simulink model "Fixed_Wing_Aircraft_Sim_closed_loop"  (R2023b)
settings: Solver=ode15s  StartTime=0.0  StopTime=10000  MinStep=1e-200  RelTol=1e-3
InitFcn:
  | parameters
undefined symbols (not defined in the file or in its folder): drawAircraft, plotmavstatevariables
settings Model: Creator=Pravin  LastModifiedBy=yizho
settings SolverCC: AlgebraicLoopSolver=TrustRegion
settings DataIOCC: ReturnWorkspaceOutputs=off
settings DebuggingCC: UnconnectedInputMsg=warning  UnconnectedOutputMsg=warning  UnconnectedLineMsg=warning  ArithmeticOperatorsInVariantConditions=warning
settings ModelReferenceCC: EnableRefExpFcnMdlSchedulingChecks=on
settings SFSimCC: SimUseLocalCustomCode=off  CustomCodeUndefinedFunction=UseInterfaceOnly
settings RTWCC: RTWUseLocalCustomCode=off  DLArmComputeVersion=19.05
settings CodeAppCC: StateflowObjectComments=on

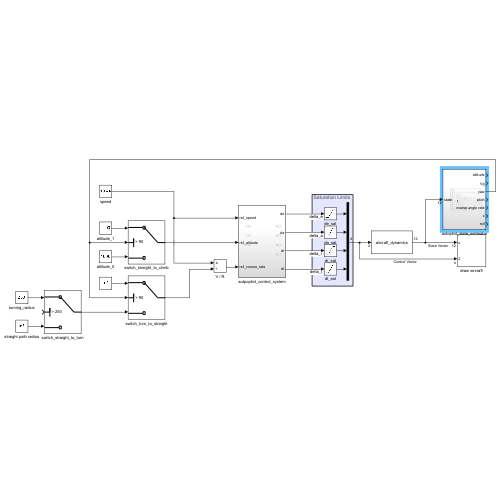
[thumbnail: Simulink's stored preview of the top-level diagram]
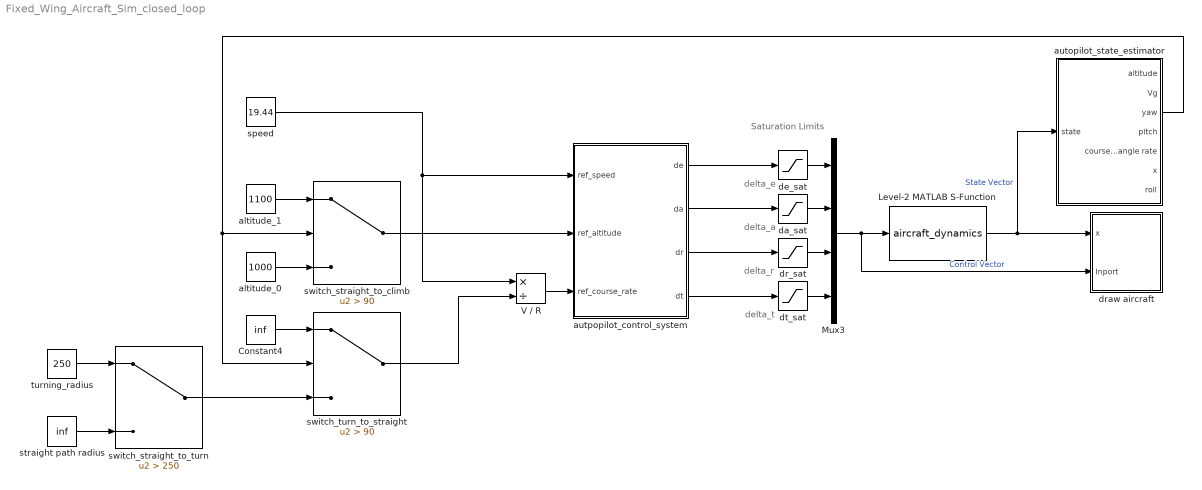
== system Fixed_Wing_Aircraft_Sim_closed_loop ==
  note: Saturation Limits
  note: delta_t
  note: delta_a
  note: delta_r
  note: delta_e
  Constant4 : Constant  Value=inf
  Level-2 MATLAB S-Function : M-S-Function  FunctionName=aircraft_dynamics  Parameters=P
  Mux3 : Mux
  V / R : Product  Inputs=*/
  altitude_0 : Constant  Value=1000
  altitude_1 : Constant  Value=1100
  autopilot_state_estimator : Subsystem
  autpopilot_control_system : Subsystem
  da_sat : Saturate  UpperLimit=50  LowerLimit=-50
  de_sat : Saturate  UpperLimit=50  LowerLimit=-50
  dr_sat : Saturate  UpperLimit=50  LowerLimit=-50
  draw aircraft : Subsystem
  dt_sat : Saturate  UpperLimit=1  LowerLimit=0
  speed : Constant  Value=19.44
  straight path radius : Constant  Value=inf
  switch_straight_to_climb : Switch  Criteria=u2 > Threshold  Threshold=90  SaturateOnIntegerOverflow=off  InputSameDT=off
  switch_straight_to_turn : Switch  Criteria=u2 > Threshold  Threshold=250  SaturateOnIntegerOverflow=off  InputSameDT=off
  switch_turn_to_straight : Switch  Criteria=u2 > Threshold  Threshold=90  SaturateOnIntegerOverflow=off  InputSameDT=off
  turning_radius : Constant  Value=250
  wires:
  Level-2 MATLAB S-Function/1 -> draw aircraft/1(x), autopilot_state_estimator/1(state)  "State Vector"
  Mux3/1 -> draw aircraft/2(Inport), Level-2 MATLAB S-Function/1  "Control Vector"
  dt_sat/1 -> Mux3/4
  de_sat/1 -> Mux3/1
  da_sat/1 -> Mux3/2
  dr_sat/1 -> Mux3/3
  switch_straight_to_turn/1 -> switch_turn_to_straight/3
  Constant4/1 -> switch_turn_to_straight/1
  straight path radius/1 -> switch_straight_to_turn/3
  turning_radius/1 -> switch_straight_to_turn/1
  altitude_1/1 -> switch_straight_to_climb/1
  altitude_0/1 -> switch_straight_to_climb/3
  speed/1 -> V / R/1, autpopilot_control_system/1(ref_speed)
  switch_straight_to_climb/1 -> autpopilot_control_system/2(ref_altitude)
  switch_turn_to_straight/1 -> V / R/2
  V / R/1 -> autpopilot_control_system/3(ref_course_rate)
  autopilot_state_estimator/3(yaw) -> switch_turn_to_straight/2, switch_straight_to_climb/2
  autpopilot_control_system/1(de) -> de_sat/1
  autpopilot_control_system/2(da) -> da_sat/1
  autpopilot_control_system/3(dr) -> dr_sat/1
  autpopilot_control_system/4(dt) -> dt_sat/1

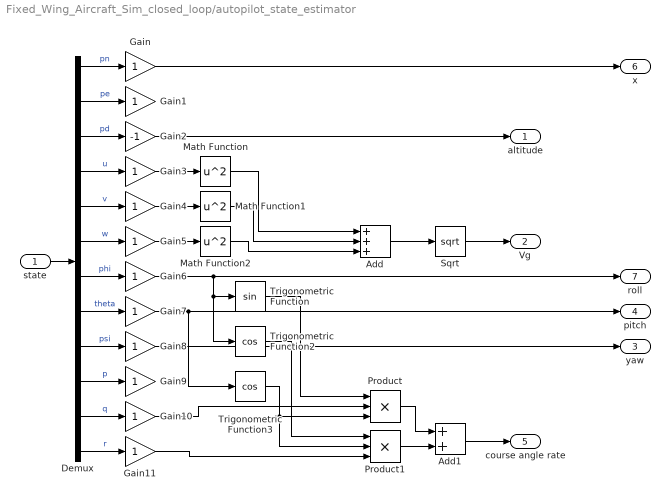
== system Fixed_Wing_Aircraft_Sim_closed_loop/autopilot_state_estimator ==
  state : Inport
  Add : Sum  Inputs=+++
  Add1 : Sum
  Demux : Demux  Outputs=12
  Gain{,1,3..11} (11 alike) : Gain
  Gain2 : Gain  Gain=-1
  Math Function : Math  Operator=square
  Math Function1 : Math  Operator=square
  Math Function2 : Math  Operator=square
  Product : Product  Inputs=3
  Product1 : Product  Inputs=3
  Sqrt : Sqrt
  Trigonometric Function : Trigonometry
  Trigonometric Function2 : Trigonometry  Operator=cos
  Trigonometric Function3 : Trigonometry  Operator=cos
  altitude : Outport
  Vg : Outport  Port=2
  yaw : Outport  Port=3
  pitch : Outport  Port=4
  course angle rate : Outport  Port=5
  x : Outport  Port=6
  roll : Outport  Port=7
  wires:
  state/1 -> Demux/1
  Demux/1 -> Gain/1  "pn"
  Demux/2 -> Gain1/1  "pe"
  Demux/3 -> Gain2/1  "pd"
  Demux/4 -> Gain3/1  "u"
  Demux/5 -> Gain4/1  "v"
  Demux/6 -> Gain5/1  "w"
  Demux/7 -> Gain6/1  "phi"
  Demux/8 -> Gain7/1  "theta"
  Demux/9 -> Gain8/1  "psi"
  Demux/10 -> Gain9/1  "p"
  Demux/11 -> Gain10/1  "q"
  Demux/12 -> Gain11/1  "r"
  Gain2/1 -> altitude/1
  Gain7/1 -> Trigonometric Function3/1, pitch/1
  Sqrt/1 -> Vg/1
  Gain3/1 -> Math Function/1
  Gain4/1 -> Math Function1/1
  Gain5/1 -> Math Function2/1
  Add/1 -> Sqrt/1
  Math Function/1 -> Add/1
  Math Function1/1 -> Add/2
  Math Function2/1 -> Add/3
  Add1/1 -> course angle rate/1
  Product/1 -> Add1/1
  Product1/1 -> Add1/2
  Gain11/1 -> Product1/3
  Gain10/1 -> Product/2
  Trigonometric Function3/1 -> Product/3, Product1/2
  Trigonometric Function2/1 -> Product1/1
  Trigonometric Function/1 -> Product/1
  Gain6/1 -> roll/1, Trigonometric Function2/1, Trigonometric Function/1
  Gain/1 -> x/1
  Gain8/1 -> yaw/1

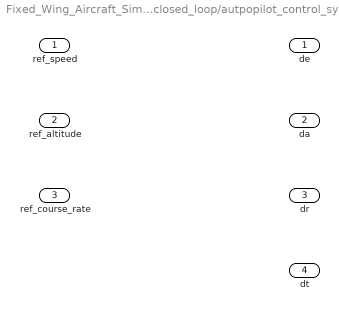
== system Fixed_Wing_Aircraft_Sim_closed_loop/autpopilot_control_system ==
  ref_speed : Inport
  ref_altitude : Inport  Port=2
  ref_course_rate : Inport  Port=3
  de : Outport
  da : Outport  Port=2
  dr : Outport  Port=3
  dt : Outport  Port=4

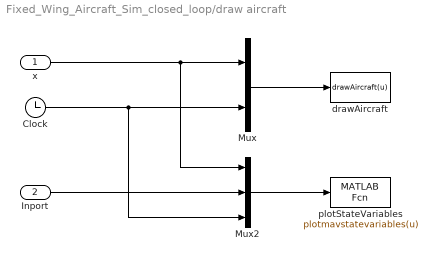
== system Fixed_Wing_Aircraft_Sim_closed_loop/draw aircraft ==
  x : Inport
  Inport : Inport  Port=2
  Clock : Clock
  Mux : Mux  Inputs=2
  Mux2 : Mux  Inputs=3
  drawAircraft : MATLABFcn  MATLABFcn=drawAircraft(u)  OutputDimensions=0  SampleTime=0.1
  plotStateVariables : MATLABFcn  MATLABFcn=plotmavstatevariables(u)  OutputDimensions=0  SampleTime=0.1
  wires:
  Clock/1 -> Mux2/3, Mux/2
  x/1 -> Mux2/1, Mux/1
  Mux/1 -> drawAircraft/1
  Mux2/1 -> plotStateVariables/1
  Inport/1 -> Mux2/2
